simulink model "DFADAS2_SenFus_v1_201204RC_training_210115"  (R2018b)
settings: Solver=FixedStepDiscrete  StartTime=0.0  StopTime=inf  FixedStep=0.002  RelTol=1e-3  EnableMultiTasking=on
PreLoadFcn:
  | RTWConfigurationCB('preloadfcn', bdroot);
libraries: canmsglib x108, simulink x48, canfdmsglib x12
(part 3 of 28)

== system DFADAS2_SenFus_v1_201204RC_training_210115/Measure Calibration Debug/CAN Monitor (CANMon)/FLRdr ==
  <FLRdr> : Inport
  Bus Selector1 : BusSelector  OutputSignals=FLRdr_bsObjInfo.M00ObjInfo,FLRdr_bsObjInfo.M01ObjInfo,FLRdr_bsObjInfo.M10ObjInfo,FLRdr_bsObjInfo.M11ObjInfo
  Bus Selector2 : BusSelector  OutputSignals=Id_S0_003,XPos_S0_003,YPos_S0_003,XVelocity_S0_003,YVelocity_S0_003,XAcc_S0_003,YAcc_S0_003
  Bus Selector3 : BusSelector  OutputSignals=Id_S0_001,XPos_S0_001,YPos_S0_001,XVelocity_S0_001,YVelocity_S0_001,XAcc_S0_001,YAcc_S0_001
  Bus Selector4 : BusSelector  OutputSignals=Id_S0_002,XPos_S0_002,YPos_S0_002,XVelocity_S0_002,YVelocity_S0_002,XAcc_S0_002,YAcc_S0_002
  Bus Selector5 : BusSelector  OutputSignals=Id_S0_004,XPos_S0_004,YPos_S0_004,XVelocity_S0_004,YVelocity_S0_004,XAcc_S0_004,YAcc_S0_004
  CAN Pack1 : canmsglib/CAN Pack  MsgList=(none)  MsgName=CAN Msg  MsgIDType=Standard (11-bit identifier)  MsgIdentifier=2000  MsgLength=8  SignalInfo=ID$0$16$1$2$1$0$1$0$-Inf$Inf$#Xpos$16$16$1$2$1$0$0.05$-400$-Inf$Inf$#Ypos$32$16$1$2$1$0$0.01$-80$-Inf$Inf$#Vx$48$16$1$2$1$0$0.01$-80$-Inf$Inf$#  NSignals=4  StartBits=str2num('[int32(0);int32(16);int32(32);int32(48)]')  SignalSizes=str2num('[int32(16);int32(16);int32(16);int32(16)]')  ByteOrders=str2num('[int32(1);int32(1);int32(1);int32(1)]')  DataTypes=str2num('[int32(2);int32(2);int32(2);int32(2)]')  MultiplexTypes=str2num('[int32(1);int32(1);int32(1);int32(1)]')  MultiplexValues=str2num('[double(0);double(0);double(0);double(0)]')  Factors=str2num('[double(1);double(0.05);double(0.01);double(0.01)]')  Offsets=str2num('[double(0);double(-400);double(-80);double(-80)]')  Minimums=str2num('[double(-Inf);double(-Inf);double(-Inf);double(-Inf)]')  Maximums=str2num('[double(Inf);double(Inf);double(Inf);double(Inf)]')  Remote=off  ApplyMinMax=off  BusOutput=on
      settings: SourceProductName=Simulink Real-Time  SourceProductBaseCode=XP  DataFormat=manually specified signals
  CAN Pack2 : canmsglib/CAN Pack  MsgList=(none)  MsgName=CAN Msg  MsgIDType=Standard (11-bit identifier)  MsgIdentifier=2001  MsgLength=8  SignalInfo=VY$0$16$1$2$1$0$0.01$-80$-Inf$Inf$#Ax$16$16$1$2$1$0$0.01$-80$-Inf$Inf$#Ay$32$16$1$2$1$0$0.01$-80$-Inf$Inf$#singal$48$16$1$2$1$0$0.01$-80$-Inf$Inf$#  NSignals=4  StartBits=str2num('[int32(0);int32(16);int32(32);int32(48)]')  SignalSizes=str2num('[int32(16);int32(16);int32(16);int32(16)]')  ByteOrders=str2num('[int32(1);int32(1);int32(1);int32(1)]')  DataTypes=str2num('[int32(2);int32(2);int32(2);int32(2)]')  MultiplexTypes=str2num('[int32(1);int32(1);int32(1);int32(1)]')  MultiplexValues=str2num('[double(0);double(0);double(0);double(0)]')  Factors=str2num('[double(0.01);double(0.01);double(0.01);double(0.01)]')  Offsets=str2num('[double(-80);double(-80);double(-80);double(-80)]')  Minimums=str2num('[double(-Inf);double(-Inf);double(-Inf);double(-Inf)]')  Maximums=str2num('[double(Inf);double(Inf);double(Inf);double(Inf)]')  Remote=off  ApplyMinMax=off  BusOutput=on
      settings: SourceProductName=Simulink Real-Time  SourceProductBaseCode=XP  DataFormat=manually specified signals
  CAN Pack3 : canmsglib/CAN Pack  MsgList=(none)  MsgName=CAN Msg  MsgIDType=Standard (11-bit identifier)  MsgIdentifier=2002  MsgLength=8  SignalInfo=ID$0$16$1$2$1$0$1$0$-Inf$Inf$#Xpos$16$16$1$2$1$0$0.05$-400$-Inf$Inf$#Ypos$32$16$1$2$1$0$0.01$-80$-Inf$Inf$#Vx$48$16$1$2$1$0$0.01$-80$-Inf$Inf$#  NSignals=4  StartBits=str2num('[int32(0);int32(16);int32(32);int32(48)]')  SignalSizes=str2num('[int32(16);int32(16);int32(16);int32(16)]')  ByteOrders=str2num('[int32(1);int32(1);int32(1);int32(1)]')  DataTypes=str2num('[int32(2);int32(2);int32(2);int32(2)]')  MultiplexTypes=str2num('[int32(1);int32(1);int32(1);int32(1)]')  MultiplexValues=str2num('[double(0);double(0);double(0);double(0)]')  Factors=str2num('[double(1);double(0.05);double(0.01);double(0.01)]')  Offsets=str2num('[double(0);double(-400);double(-80);double(-80)]')  Minimums=str2num('[double(-Inf);double(-Inf);double(-Inf);double(-Inf)]')  Maximums=str2num('[double(Inf);double(Inf);double(Inf);double(Inf)]')  Remote=off  ApplyMinMax=off  BusOutput=on
      settings: SourceProductName=Simulink Real-Time  SourceProductBaseCode=XP  DataFormat=manually specified signals
  CAN Pack4 : canmsglib/CAN Pack  MsgList=(none)  MsgName=CAN Msg  MsgIDType=Standard (11-bit identifier)  MsgIdentifier=2003  MsgLength=8  SignalInfo=VY$0$16$1$2$1$0$0.01$-80$-Inf$Inf$#Ax$16$16$1$2$1$0$0.01$-80$-Inf$Inf$#Ay$32$16$1$2$1$0$0.01$-80$-Inf$Inf$#singal$48$16$1$2$1$0$0.01$-80$-Inf$Inf$#  NSignals=4  StartBits=str2num('[int32(0);int32(16);int32(32);int32(48)]')  SignalSizes=str2num('[int32(16);int32(16);int32(16);int32(16)]')  ByteOrders=str2num('[int32(1);int32(1);int32(1);int32(1)]')  DataTypes=str2num('[int32(2);int32(2);int32(2);int32(2)]')  MultiplexTypes=str2num('[int32(1);int32(1);int32(1);int32(1)]')  MultiplexValues=str2num('[double(0);double(0);double(0);double(0)]')  Factors=str2num('[double(0.01);double(0.01);double(0.01);double(0.01)]')  Offsets=str2num('[double(-80);double(-80);double(-80);double(-80)]')  Minimums=str2num('[double(-Inf);double(-Inf);double(-Inf);double(-Inf)]')  Maximums=str2num('[double(Inf);double(Inf);double(Inf);double(Inf)]')  Remote=off  ApplyMinMax=off  BusOutput=on
      settings: SourceProductName=Simulink Real-Time  SourceProductBaseCode=XP  DataFormat=manually specified signals
  CAN Pack5 : canmsglib/CAN Pack  MsgList=(none)  MsgName=CAN Msg  MsgIDType=Standard (11-bit identifier)  MsgIdentifier=2004  MsgLength=8  SignalInfo=ID$0$16$1$2$1$0$1$0$-Inf$Inf$#Xpos$16$16$1$2$1$0$0.05$-400$-Inf$Inf$#Ypos$32$16$1$2$1$0$0.01$-80$-Inf$Inf$#Vx$48$16$1$2$1$0$0.01$-80$-Inf$Inf$#  NSignals=4  StartBits=str2num('[int32(0);int32(16);int32(32);int32(48)]')  SignalSizes=str2num('[int32(16);int32(16);int32(16);int32(16)]')  ByteOrders=str2num('[int32(1);int32(1);int32(1);int32(1)]')  DataTypes=str2num('[int32(2);int32(2);int32(2);int32(2)]')  MultiplexTypes=str2num('[int32(1);int32(1);int32(1);int32(1)]')  MultiplexValues=str2num('[double(0);double(0);double(0);double(0)]')  Factors=str2num('[double(1);double(0.05);double(0.01);double(0.01)]')  Offsets=str2num('[double(0);double(-400);double(-80);double(-80)]')  Minimums=str2num('[double(-Inf);double(-Inf);double(-Inf);double(-Inf)]')  Maximums=str2num('[double(Inf);double(Inf);double(Inf);double(Inf)]')  Remote=off  ApplyMinMax=off  BusOutput=on
      settings: SourceProductName=Simulink Real-Time  SourceProductBaseCode=XP  DataFormat=manually specified signals
  CAN Pack6 : canmsglib/CAN Pack  MsgList=(none)  MsgName=CAN Msg  MsgIDType=Standard (11-bit identifier)  MsgIdentifier=2005  MsgLength=8  SignalInfo=VY$0$16$1$2$1$0$0.01$-80$-Inf$Inf$#Ax$16$16$1$2$1$0$0.01$-80$-Inf$Inf$#Ay$32$16$1$2$1$0$0.01$-80$-Inf$Inf$#singal$48$16$1$2$1$0$0.01$-80$-Inf$Inf$#  NSignals=4  StartBits=str2num('[int32(0);int32(16);int32(32);int32(48)]')  SignalSizes=str2num('[int32(16);int32(16);int32(16);int32(16)]')  ByteOrders=str2num('[int32(1);int32(1);int32(1);int32(1)]')  DataTypes=str2num('[int32(2);int32(2);int32(2);int32(2)]')  MultiplexTypes=str2num('[int32(1);int32(1);int32(1);int32(1)]')  MultiplexValues=str2num('[double(0);double(0);double(0);double(0)]')  Factors=str2num('[double(0.01);double(0.01);double(0.01);double(0.01)]')  Offsets=str2num('[double(-80);double(-80);double(-80);double(-80)]')  Minimums=str2num('[double(-Inf);double(-Inf);double(-Inf);double(-Inf)]')  Maximums=str2num('[double(Inf);double(Inf);double(Inf);double(Inf)]')  Remote=off  ApplyMinMax=off  BusOutput=on
      settings: SourceProductName=Simulink Real-Time  SourceProductBaseCode=XP  DataFormat=manually specified signals
  CAN Pack7 : canmsglib/CAN Pack  MsgList=(none)  MsgName=CAN Msg  MsgIDType=Standard (11-bit identifier)  MsgIdentifier=2006  MsgLength=8  SignalInfo=ID$0$16$1$2$1$0$1$0$-Inf$Inf$#Xpos$16$16$1$2$1$0$0.05$-400$-Inf$Inf$#Ypos$32$16$1$2$1$0$0.01$-80$-Inf$Inf$#Vx$48$16$1$2$1$0$0.01$-80$-Inf$Inf$#  NSignals=4  StartBits=str2num('[int32(0);int32(16);int32(32);int32(48)]')  SignalSizes=str2num('[int32(16);int32(16);int32(16);int32(16)]')  ByteOrders=str2num('[int32(1);int32(1);int32(1);int32(1)]')  DataTypes=str2num('[int32(2);int32(2);int32(2);int32(2)]')  MultiplexTypes=str2num('[int32(1);int32(1);int32(1);int32(1)]')  MultiplexValues=str2num('[double(0);double(0);double(0);double(0)]')  Factors=str2num('[double(1);double(0.05);double(0.01);double(0.01)]')  Offsets=str2num('[double(0);double(-400);double(-80);double(-80)]')  Minimums=str2num('[double(-Inf);double(-Inf);double(-Inf);double(-Inf)]')  Maximums=str2num('[double(Inf);double(Inf);double(Inf);double(Inf)]')  Remote=off  ApplyMinMax=off  BusOutput=on
      settings: SourceProductName=Simulink Real-Time  SourceProductBaseCode=XP  DataFormat=manually specified signals
  CAN Pack8 : canmsglib/CAN Pack  MsgList=(none)  MsgName=CAN Msg  MsgIDType=Standard (11-bit identifier)  MsgIdentifier=2007  MsgLength=8  SignalInfo=VY$0$16$1$2$1$0$0.01$-80$-Inf$Inf$#Ax$16$16$1$2$1$0$0.01$-80$-Inf$Inf$#Ay$32$16$1$2$1$0$0.01$-80$-Inf$Inf$#singal$48$16$1$2$1$0$0.01$-80$-Inf$Inf$#  NSignals=4  StartBits=str2num('[int32(0);int32(16);int32(32);int32(48)]')  SignalSizes=str2num('[int32(16);int32(16);int32(16);int32(16)]')  ByteOrders=str2num('[int32(1);int32(1);int32(1);int32(1)]')  DataTypes=str2num('[int32(2);int32(2);int32(2);int32(2)]')  MultiplexTypes=str2num('[int32(1);int32(1);int32(1);int32(1)]')  MultiplexValues=str2num('[double(0);double(0);double(0);double(0)]')  Factors=str2num('[double(0.01);double(0.01);double(0.01);double(0.01)]')  Offsets=str2num('[double(-80);double(-80);double(-80);double(-80)]')  Minimums=str2num('[double(-Inf);double(-Inf);double(-Inf);double(-Inf)]')  Maximums=str2num('[double(Inf);double(Inf);double(Inf);double(Inf)]')  Remote=off  ApplyMinMax=off  BusOutput=on
      settings: SourceProductName=Simulink Real-Time  SourceProductBaseCode=XP  DataFormat=manually specified signals
  S-Function1 : S-Function  FunctionName=NSTC297CANTransmitBlkLib  Parameters=|  SFunctionDeploymentMode=off  EnableBusSupport=off  mask(NSTC297 CAN Transmit){Ns_DeviceID=General Control Unit Gen2, Ns_ChannelNum=0, Ns_FrameType=CAN, Ns_FrameBufferSize=0, Ns_OverflowCntOutFlg=off, Ns_SampleTime=-1}
      | uint16(Ns_DeviceID),
      | uint16(Ns_ChannelNum),
      | uint16(Ns_FrameType),
      | uint16(Ns_FrameBufferSize),
      | uint8(Ns_OverflowCntOutFlg),
      | double(Ns_SampleTime)
      mask prompts: Ns_DeviceID "Device:"; Ns_ChannelNum "Channel number:"; Ns_FrameType "Frame type:"; Ns_FrameBufferSize "Frame buffer size:"; Ns_OverflowCntOutFlg "Overflow count output"; Ns_SampleTime "Sample time:"
      mask init:
      | NSTC297CANTransmit_callback('portlabels');
      mask TypeOptions Ns_DeviceID: General Control Unit Gen2 | ADAS Control Unit Gen2
      mask TypeOptions Ns_ChannelNum: 0 | 1 | 2 | 3 | 4 | 5
      mask TypeOptions Ns_FrameType: CAN | CANFD
      mask Display: color('blue');text(0.98,0.9,'NovSteeds TC297','horizontalAlignment','right');color('blue');text(0.5,0.65,'CAN Transmit','horizontalAlignment','center');color('black');text(0.5,0.35,'Type: CAN','horizontalAlignment','center');text(0.5,0.50,'Channel: 0','horizontalAlignment','center');port_label('input',1, 'Msg');
  S-Function2 : S-Function  FunctionName=NSTC297CANTransmitBlkLib  Parameters=|  SFunctionDeploymentMode=off  EnableBusSupport=off  mask(NSTC297 CAN Transmit){Ns_DeviceID=General Control Unit Gen2, Ns_ChannelNum=0, Ns_FrameType=CAN, Ns_FrameBufferSize=0, Ns_OverflowCntOutFlg=off, Ns_SampleTime=-1}
      | uint16(Ns_DeviceID),
      | uint16(Ns_ChannelNum),
      | uint16(Ns_FrameType),
      | uint16(Ns_FrameBufferSize),
      | uint8(Ns_OverflowCntOutFlg),
      | double(Ns_SampleTime)
      mask prompts: Ns_DeviceID "Device:"; Ns_ChannelNum "Channel number:"; Ns_FrameType "Frame type:"; Ns_FrameBufferSize "Frame buffer size:"; Ns_OverflowCntOutFlg "Overflow count output"; Ns_SampleTime "Sample time:"
      mask init:
      | NSTC297CANTransmit_callback('portlabels');
      mask TypeOptions Ns_DeviceID: General Control Unit Gen2 | ADAS Control Unit Gen2
      mask TypeOptions Ns_ChannelNum: 0 | 1 | 2 | 3 | 4 | 5
      mask TypeOptions Ns_FrameType: CAN | CANFD
      mask Display: color('blue');text(0.98,0.9,'NovSteeds TC297','horizontalAlignment','right');color('blue');text(0.5,0.65,'CAN Transmit','horizontalAlignment','center');color('black');text(0.5,0.35,'Type: CAN','horizontalAlignment','center');text(0.5,0.50,'Channel: 0','horizontalAlignment','center');port_label('input',1, 'Msg');
  S-Function3 : S-Function  FunctionName=NSTC297CANTransmitBlkLib  Parameters=|  SFunctionDeploymentMode=off  EnableBusSupport=off  mask(NSTC297 CAN Transmit){Ns_DeviceID=General Control Unit Gen2, Ns_ChannelNum=0, Ns_FrameType=CAN, Ns_FrameBufferSize=0, Ns_OverflowCntOutFlg=off, Ns_SampleTime=-1}
      | uint16(Ns_DeviceID),
      | uint16(Ns_ChannelNum),
      | uint16(Ns_FrameType),
      | uint16(Ns_FrameBufferSize),
      | uint8(Ns_OverflowCntOutFlg),
      | double(Ns_SampleTime)
      mask prompts: Ns_DeviceID "Device:"; Ns_ChannelNum "Channel number:"; Ns_FrameType "Frame type:"; Ns_FrameBufferSize "Frame buffer size:"; Ns_OverflowCntOutFlg "Overflow count output"; Ns_SampleTime "Sample time:"
      mask init:
      | NSTC297CANTransmit_callback('portlabels');
      mask TypeOptions Ns_DeviceID: General Control Unit Gen2 | ADAS Control Unit Gen2
      mask TypeOptions Ns_ChannelNum: 0 | 1 | 2 | 3 | 4 | 5
      mask TypeOptions Ns_FrameType: CAN | CANFD
      mask Display: color('blue');text(0.98,0.9,'NovSteeds TC297','horizontalAlignment','right');color('blue');text(0.5,0.65,'CAN Transmit','horizontalAlignment','center');color('black');text(0.5,0.35,'Type: CAN','horizontalAlignment','center');text(0.5,0.50,'Channel: 0','horizontalAlignment','center');port_label('input',1, 'Msg');
  S-Function4 : S-Function  FunctionName=NSTC297CANTransmitBlkLib  Parameters=|  SFunctionDeploymentMode=off  EnableBusSupport=off  mask(NSTC297 CAN Transmit){Ns_DeviceID=General Control Unit Gen2, Ns_ChannelNum=0, Ns_FrameType=CAN, Ns_FrameBufferSize=0, Ns_OverflowCntOutFlg=off, Ns_SampleTime=-1}
      | uint16(Ns_DeviceID),
      | uint16(Ns_ChannelNum),
      | uint16(Ns_FrameType),
      | uint16(Ns_FrameBufferSize),
      | uint8(Ns_OverflowCntOutFlg),
      | double(Ns_SampleTime)
      mask prompts: Ns_DeviceID "Device:"; Ns_ChannelNum "Channel number:"; Ns_FrameType "Frame type:"; Ns_FrameBufferSize "Frame buffer size:"; Ns_OverflowCntOutFlg "Overflow count output"; Ns_SampleTime "Sample time:"
      mask init:
      | NSTC297CANTransmit_callback('portlabels');
      mask TypeOptions Ns_DeviceID: General Control Unit Gen2 | ADAS Control Unit Gen2
      mask TypeOptions Ns_ChannelNum: 0 | 1 | 2 | 3 | 4 | 5
      mask TypeOptions Ns_FrameType: CAN | CANFD
      mask Display: color('blue');text(0.98,0.9,'NovSteeds TC297','horizontalAlignment','right');color('blue');text(0.5,0.65,'CAN Transmit','horizontalAlignment','center');color('black');text(0.5,0.35,'Type: CAN','horizontalAlignment','center');text(0.5,0.50,'Channel: 0','horizontalAlignment','center');port_label('input',1, 'Msg');
  S-Function5 : S-Function  FunctionName=NSTC297CANTransmitBlkLib  Parameters=|  SFunctionDeploymentMode=off  EnableBusSupport=off  mask(NSTC297 CAN Transmit){Ns_DeviceID=General Control Unit Gen2, Ns_ChannelNum=0, Ns_FrameType=CAN, Ns_FrameBufferSize=0, Ns_OverflowCntOutFlg=off, Ns_SampleTime=-1}
      | uint16(Ns_DeviceID),
      | uint16(Ns_ChannelNum),
      | uint16(Ns_FrameType),
      | uint16(Ns_FrameBufferSize),
      | uint8(Ns_OverflowCntOutFlg),
      | double(Ns_SampleTime)
      mask prompts: Ns_DeviceID "Device:"; Ns_ChannelNum "Channel number:"; Ns_FrameType "Frame type:"; Ns_FrameBufferSize "Frame buffer size:"; Ns_OverflowCntOutFlg "Overflow count output"; Ns_SampleTime "Sample time:"
      mask init:
      | NSTC297CANTransmit_callback('portlabels');
      mask TypeOptions Ns_DeviceID: General Control Unit Gen2 | ADAS Control Unit Gen2
      mask TypeOptions Ns_ChannelNum: 0 | 1 | 2 | 3 | 4 | 5
      mask TypeOptions Ns_FrameType: CAN | CANFD
      mask Display: color('blue');text(0.98,0.9,'NovSteeds TC297','horizontalAlignment','right');color('blue');text(0.5,0.65,'CAN Transmit','horizontalAlignment','center');color('black');text(0.5,0.35,'Type: CAN','horizontalAlignment','center');text(0.5,0.50,'Channel: 0','horizontalAlignment','center');port_label('input',1, 'Msg');
  S-Function6 : S-Function  FunctionName=NSTC297CANTransmitBlkLib  Parameters=|  SFunctionDeploymentMode=off  EnableBusSupport=off  mask(NSTC297 CAN Transmit){Ns_DeviceID=General Control Unit Gen2, Ns_ChannelNum=0, Ns_FrameType=CAN, Ns_FrameBufferSize=0, Ns_OverflowCntOutFlg=off, Ns_SampleTime=-1}
      | uint16(Ns_DeviceID),
      | uint16(Ns_ChannelNum),
      | uint16(Ns_FrameType),
      | uint16(Ns_FrameBufferSize),
      | uint8(Ns_OverflowCntOutFlg),
      | double(Ns_SampleTime)
      mask prompts: Ns_DeviceID "Device:"; Ns_ChannelNum "Channel number:"; Ns_FrameType "Frame type:"; Ns_FrameBufferSize "Frame buffer size:"; Ns_OverflowCntOutFlg "Overflow count output"; Ns_SampleTime "Sample time:"
      mask init:
      | NSTC297CANTransmit_callback('portlabels');
      mask TypeOptions Ns_DeviceID: General Control Unit Gen2 | ADAS Control Unit Gen2
      mask TypeOptions Ns_ChannelNum: 0 | 1 | 2 | 3 | 4 | 5
      mask TypeOptions Ns_FrameType: CAN | CANFD
      mask Display: color('blue');text(0.98,0.9,'NovSteeds TC297','horizontalAlignment','right');color('blue');text(0.5,0.65,'CAN Transmit','horizontalAlignment','center');color('black');text(0.5,0.35,'Type: CAN','horizontalAlignment','center');text(0.5,0.50,'Channel: 0','horizontalAlignment','center');port_label('input',1, 'Msg');
  S-Function7 : S-Function  FunctionName=NSTC297CANTransmitBlkLib  Parameters=|  SFunctionDeploymentMode=off  EnableBusSupport=off  mask(NSTC297 CAN Transmit){Ns_DeviceID=General Control Unit Gen2, Ns_ChannelNum=0, Ns_FrameType=CAN, Ns_FrameBufferSize=0, Ns_OverflowCntOutFlg=off, Ns_SampleTime=-1}
      | uint16(Ns_DeviceID),
      | uint16(Ns_ChannelNum),
      | uint16(Ns_FrameType),
      | uint16(Ns_FrameBufferSize),
      | uint8(Ns_OverflowCntOutFlg),
      | double(Ns_SampleTime)
      mask prompts: Ns_DeviceID "Device:"; Ns_ChannelNum "Channel number:"; Ns_FrameType "Frame type:"; Ns_FrameBufferSize "Frame buffer size:"; Ns_OverflowCntOutFlg "Overflow count output"; Ns_SampleTime "Sample time:"
      mask init:
      | NSTC297CANTransmit_callback('portlabels');
      mask TypeOptions Ns_DeviceID: General Control Unit Gen2 | ADAS Control Unit Gen2
      mask TypeOptions Ns_ChannelNum: 0 | 1 | 2 | 3 | 4 | 5
      mask TypeOptions Ns_FrameType: CAN | CANFD
      mask Display: color('blue');text(0.98,0.9,'NovSteeds TC297','horizontalAlignment','right');color('blue');text(0.5,0.65,'CAN Transmit','horizontalAlignment','center');color('black');text(0.5,0.35,'Type: CAN','horizontalAlignment','center');text(0.5,0.50,'Channel: 0','horizontalAlignment','center');port_label('input',1, 'Msg');
  S-Function8 : S-Function  FunctionName=NSTC297CANTransmitBlkLib  Parameters=|  SFunctionDeploymentMode=off  EnableBusSupport=off  mask(NSTC297 CAN Transmit){Ns_DeviceID=General Control Unit Gen2, Ns_ChannelNum=0, Ns_FrameType=CAN, Ns_FrameBufferSize=0, Ns_OverflowCntOutFlg=off, Ns_SampleTime=-1}
      | uint16(Ns_DeviceID),
      | uint16(Ns_ChannelNum),
      | uint16(Ns_FrameType),
      | uint16(Ns_FrameBufferSize),
      | uint8(Ns_OverflowCntOutFlg),
      | double(Ns_SampleTime)
      mask prompts: Ns_DeviceID "Device:"; Ns_ChannelNum "Channel number:"; Ns_FrameType "Frame type:"; Ns_FrameBufferSize "Frame buffer size:"; Ns_OverflowCntOutFlg "Overflow count output"; Ns_SampleTime "Sample time:"
      mask init:
      | NSTC297CANTransmit_callback('portlabels');
      mask TypeOptions Ns_DeviceID: General Control Unit Gen2 | ADAS Control Unit Gen2
      mask TypeOptions Ns_ChannelNum: 0 | 1 | 2 | 3 | 4 | 5
      mask TypeOptions Ns_FrameType: CAN | CANFD
      mask Display: color('blue');text(0.98,0.9,'NovSteeds TC297','horizontalAlignment','right');color('blue');text(0.5,0.65,'CAN Transmit','horizontalAlignment','center');color('black');text(0.5,0.35,'Type: CAN','horizontalAlignment','center');text(0.5,0.50,'Channel: 0','horizontalAlignment','center');port_label('input',1, 'Msg');
  wires:
  Bus Selector1/1 -> Bus Selector3/1  "<M00ObjInfo>"
  Bus Selector1/2 -> Bus Selector4/1  "<M01ObjInfo>"
  Bus Selector1/4 -> Bus Selector5/1  "<M11ObjInfo>"
  Bus Selector1/3 -> Bus Selector2/1  "<M10ObjInfo>"
  <FLRdr>/1 -> Bus Selector1/1
  CAN Pack1/1 -> S-Function8/1
  CAN Pack2/1 -> S-Function1/1
  Bus Selector3/5 -> CAN Pack2/1  "<YVelocity_S0_001>"
  Bus Selector3/6 -> CAN Pack2/2  "<XAcc_S0_001>"
  Bus Selector3/7 -> CAN Pack2/3  "<YAcc_S0_001>"
  Bus Selector3/1 -> CAN Pack1/1  "<Id_S0_001>"
  Bus Selector3/2 -> CAN Pack1/2  "<XPos_S0_001>"
  Bus Selector3/3 -> CAN Pack1/3  "<YPos_S0_001>"
  Bus Selector3/4 -> CAN Pack1/4  "<XVelocity_S0_001>"
  Bus Selector4/4 -> CAN Pack3/4  "<XVelocity_S0_002>"
  Bus Selector4/3 -> CAN Pack3/3  "<YPos_S0_002>"
  Bus Selector4/2 -> CAN Pack3/2  "<XPos_S0_002>"
  Bus Selector4/1 -> CAN Pack3/1  "<Id_S0_002>"
  Bus Selector4/7 -> CAN Pack4/3  "<YAcc_S0_002>"
  Bus Selector4/6 -> CAN Pack4/2  "<XAcc_S0_002>"
  Bus Selector4/5 -> CAN Pack4/1  "<YVelocity_S0_002>"
  CAN Pack4/1 -> S-Function2/1
  CAN Pack3/1 -> S-Function3/1
  CAN Pack5/1 -> S-Function5/1
  CAN Pack6/1 -> S-Function4/1
  Bus Selector2/5 -> CAN Pack6/1  "<YVelocity_S0_003>"
  Bus Selector2/6 -> CAN Pack6/2  "<XAcc_S0_003>"
  Bus Selector2/7 -> CAN Pack6/3  "<YAcc_S0_003>"
  Bus Selector2/1 -> CAN Pack5/1  "<Id_S0_003>"
  Bus Selector2/2 -> CAN Pack5/2  "<XPos_S0_003>"
  Bus Selector2/3 -> CAN Pack5/3  "<YPos_S0_003>"
  Bus Selector2/4 -> CAN Pack5/4  "<XVelocity_S0_003>"
  Bus Selector5/4 -> CAN Pack7/4  "<XVelocity_S0_004>"
  Bus Selector5/3 -> CAN Pack7/3  "<YPos_S0_004>"
  Bus Selector5/2 -> CAN Pack7/2  "<XPos_S0_004>"
  Bus Selector5/7 -> CAN Pack8/3  "<YAcc_S0_004>"
  Bus Selector5/6 -> CAN Pack8/2  "<XAcc_S0_004>"
  Bus Selector5/5 -> CAN Pack8/1  "<YVelocity_S0_004>"
  CAN Pack8/1 -> S-Function6/1
  CAN Pack7/1 -> S-Function7/1
  Bus Selector5/1 -> CAN Pack7/1  "<Id_S0_004>"

== system DFADAS2_SenFus_v1_201204RC_training_210115/Measure Calibration Debug/CAN Monitor (CANMon)/FRRdr ==
  <FRRdr> : Inport
  Bus Selector1 : BusSelector  OutputSignals=FRRdr_bsObjInfo.M00ObjInfo,FRRdr_bsObjInfo.M01ObjInfo,FRRdr_bsObjInfo.M10ObjInfo,FRRdr_bsObjInfo.M11ObjInfo
  Bus Selector2 : BusSelector  OutputSignals=Id_S0_003,XPos_S0_003,YPos_S0_003,XVelocity_S0_003,YVelocity_S0_003,XAcc_S0_003,YAcc_S0_003
  Bus Selector3 : BusSelector  OutputSignals=Id_S0_001,XPos_S0_001,YPos_S0_001,XVelocity_S0_001,YVelocity_S0_001,XAcc_S0_001,YAcc_S0_001
  Bus Selector4 : BusSelector  OutputSignals=Id_S0_002,XPos_S0_002,YPos_S0_002,XVelocity_S0_002,YVelocity_S0_002,XAcc_S0_002,YAcc_S0_002
  Bus Selector5 : BusSelector  OutputSignals=Id_S0_004,XPos_S0_004,YPos_S0_004,XVelocity_S0_004,YVelocity_S0_004,XAcc_S0_004,YAcc_S0_004
  CAN Pack1 : canmsglib/CAN Pack  MsgList=(none)  MsgName=CAN Msg  MsgIDType=Standard (11-bit identifier)  MsgIdentifier=2008  MsgLength=8  SignalInfo=ID$0$16$1$2$1$0$1$0$-Inf$Inf$#Xpos$16$16$1$2$1$0$0.05$-400$-Inf$Inf$#Ypos$32$16$1$2$1$0$0.01$-80$-Inf$Inf$#Vx$48$16$1$2$1$0$0.01$-80$-Inf$Inf$#  NSignals=4  StartBits=str2num('[int32(0);int32(16);int32(32);int32(48)]')  SignalSizes=str2num('[int32(16);int32(16);int32(16);int32(16)]')  ByteOrders=str2num('[int32(1);int32(1);int32(1);int32(1)]')  DataTypes=str2num('[int32(2);int32(2);int32(2);int32(2)]')  MultiplexTypes=str2num('[int32(1);int32(1);int32(1);int32(1)]')  MultiplexValues=str2num('[double(0);double(0);double(0);double(0)]')  Factors=str2num('[double(1);double(0.05);double(0.01);double(0.01)]')  Offsets=str2num('[double(0);double(-400);double(-80);double(-80)]')  Minimums=str2num('[double(-Inf);double(-Inf);double(-Inf);double(-Inf)]')  Maximums=str2num('[double(Inf);double(Inf);double(Inf);double(Inf)]')  Remote=off  ApplyMinMax=off  BusOutput=on
      settings: SourceProductName=Simulink Real-Time  SourceProductBaseCode=XP  DataFormat=manually specified signals
  CAN Pack10 : canmsglib/CAN Pack  MsgList=(none)  MsgName=CAN Msg  MsgIDType=Standard (11-bit identifier)  MsgIdentifier=2015  MsgLength=8  SignalInfo=VY$0$16$1$2$1$0$0.01$-80$-Inf$Inf$#Ax$16$16$1$2$1$0$0.01$-80$-Inf$Inf$#Ay$32$16$1$2$1$0$0.01$-80$-Inf$Inf$#singal$48$16$1$2$1$0$0.01$-80$-Inf$Inf$#  NSignals=4  StartBits=str2num('[int32(0);int32(16);int32(32);int32(48)]')  SignalSizes=str2num('[int32(16);int32(16);int32(16);int32(16)]')  ByteOrders=str2num('[int32(1);int32(1);int32(1);int32(1)]')  DataTypes=str2num('[int32(2);int32(2);int32(2);int32(2)]')  MultiplexTypes=str2num('[int32(1);int32(1);int32(1);int32(1)]')  MultiplexValues=str2num('[double(0);double(0);double(0);double(0)]')  Factors=str2num('[double(0.01);double(0.01);double(0.01);double(0.01)]')  Offsets=str2num('[double(-80);double(-80);double(-80);double(-80)]')  Minimums=str2num('[double(-Inf);double(-Inf);double(-Inf);double(-Inf)]')  Maximums=str2num('[double(Inf);double(Inf);double(Inf);double(Inf)]')  Remote=off  ApplyMinMax=off  BusOutput=on
      settings: SourceProductName=Simulink Real-Time  SourceProductBaseCode=XP  DataFormat=manually specified signals
  CAN Pack2 : canmsglib/CAN Pack  MsgList=(none)  MsgName=CAN Msg  MsgIDType=Standard (11-bit identifier)  MsgIdentifier=2009  MsgLength=8  SignalInfo=VY$0$16$1$2$1$0$0.01$-80$-Inf$Inf$#Ax$16$16$1$2$1$0$0.01$-80$-Inf$Inf$#Ay$32$16$1$2$1$0$0.01$-80$-Inf$Inf$#singal$48$16$1$2$1$0$0.01$-80$-Inf$Inf$#  NSignals=4  StartBits=str2num('[int32(0);int32(16);int32(32);int32(48)]')  SignalSizes=str2num('[int32(16);int32(16);int32(16);int32(16)]')  ByteOrders=str2num('[int32(1);int32(1);int32(1);int32(1)]')  DataTypes=str2num('[int32(2);int32(2);int32(2);int32(2)]')  MultiplexTypes=str2num('[int32(1);int32(1);int32(1);int32(1)]')  MultiplexValues=str2num('[double(0);double(0);double(0);double(0)]')  Factors=str2num('[double(0.01);double(0.01);double(0.01);double(0.01)]')  Offsets=str2num('[double(-80);double(-80);double(-80);double(-80)]')  Minimums=str2num('[double(-Inf);double(-Inf);double(-Inf);double(-Inf)]')  Maximums=str2num('[double(Inf);double(Inf);double(Inf);double(Inf)]')  Remote=off  ApplyMinMax=off  BusOutput=on
      settings: SourceProductName=Simulink Real-Time  SourceProductBaseCode=XP  DataFormat=manually specified signals
  CAN Pack3 : canmsglib/CAN Pack  MsgList=(none)  MsgName=CAN Msg  MsgIDType=Standard (11-bit identifier)  MsgIdentifier=2010  MsgLength=8  SignalInfo=ID$0$16$1$2$1$0$1$0$-Inf$Inf$#Xpos$16$16$1$2$1$0$0.05$-400$-Inf$Inf$#Ypos$32$16$1$2$1$0$0.01$-80$-Inf$Inf$#Vx$48$16$1$2$1$0$0.01$-80$-Inf$Inf$#  NSignals=4  StartBits=str2num('[int32(0);int32(16);int32(32);int32(48)]')  SignalSizes=str2num('[int32(16);int32(16);int32(16);int32(16)]')  ByteOrders=str2num('[int32(1);int32(1);int32(1);int32(1)]')  DataTypes=str2num('[int32(2);int32(2);int32(2);int32(2)]')  MultiplexTypes=str2num('[int32(1);int32(1);int32(1);int32(1)]')  MultiplexValues=str2num('[double(0);double(0);double(0);double(0)]')  Factors=str2num('[double(1);double(0.05);double(0.01);double(0.01)]')  Offsets=str2num('[double(0);double(-400);double(-80);double(-80)]')  Minimums=str2num('[double(-Inf);double(-Inf);double(-Inf);double(-Inf)]')  Maximums=str2num('[double(Inf);double(Inf);double(Inf);double(Inf)]')  Remote=off  ApplyMinMax=off  BusOutput=on
      settings: SourceProductName=Simulink Real-Time  SourceProductBaseCode=XP  DataFormat=manually specified signals
  CAN Pack4 : canmsglib/CAN Pack  MsgList=(none)  MsgName=CAN Msg  MsgIDType=Standard (11-bit identifier)  MsgIdentifier=2011  MsgLength=8  SignalInfo=VY$0$16$1$2$1$0$0.01$-80$-Inf$Inf$#Ax$16$16$1$2$1$0$0.01$-80$-Inf$Inf$#Ay$32$16$1$2$1$0$0.01$-80$-Inf$Inf$#singal$48$16$1$2$1$0$0.01$-80$-Inf$Inf$#  NSignals=4  StartBits=str2num('[int32(0);int32(16);int32(32);int32(48)]')  SignalSizes=str2num('[int32(16);int32(16);int32(16);int32(16)]')  ByteOrders=str2num('[int32(1);int32(1);int32(1);int32(1)]')  DataTypes=str2num('[int32(2);int32(2);int32(2);int32(2)]')  MultiplexTypes=str2num('[int32(1);int32(1);int32(1);int32(1)]')  MultiplexValues=str2num('[double(0);double(0);double(0);double(0)]')  Factors=str2num('[double(0.01);double(0.01);double(0.01);double(0.01)]')  Offsets=str2num('[double(-80);double(-80);double(-80);double(-80)]')  Minimums=str2num('[double(-Inf);double(-Inf);double(-Inf);double(-Inf)]')  Maximums=str2num('[double(Inf);double(Inf);double(Inf);double(Inf)]')  Remote=off  ApplyMinMax=off  BusOutput=on
      settings: SourceProductName=Simulink Real-Time  SourceProductBaseCode=XP  DataFormat=manually specified signals
  CAN Pack5 : canmsglib/CAN Pack  MsgList=(none)  MsgName=CAN Msg  MsgIDType=Standard (11-bit identifier)  MsgIdentifier=2012  MsgLength=8  SignalInfo=ID$0$16$1$2$1$0$1$0$-Inf$Inf$#Xpos$16$16$1$2$1$0$0.05$-400$-Inf$Inf$#Ypos$32$16$1$2$1$0$0.01$-80$-Inf$Inf$#Vx$48$16$1$2$1$0$0.01$-80$-Inf$Inf$#  NSignals=4  StartBits=str2num('[int32(0);int32(16);int32(32);int32(48)]')  SignalSizes=str2num('[int32(16);int32(16);int32(16);int32(16)]')  ByteOrders=str2num('[int32(1);int32(1);int32(1);int32(1)]')  DataTypes=str2num('[int32(2);int32(2);int32(2);int32(2)]')  MultiplexTypes=str2num('[int32(1);int32(1);int32(1);int32(1)]')  MultiplexValues=str2num('[double(0);double(0);double(0);double(0)]')  Factors=str2num('[double(1);double(0.05);double(0.01);double(0.01)]')  Offsets=str2num('[double(0);double(-400);double(-80);double(-80)]')  Minimums=str2num('[double(-Inf);double(-Inf);double(-Inf);double(-Inf)]')  Maximums=str2num('[double(Inf);double(Inf);double(Inf);double(Inf)]')  Remote=off  ApplyMinMax=off  BusOutput=on
      settings: SourceProductName=Simulink Real-Time  SourceProductBaseCode=XP  DataFormat=manually specified signals
  CAN Pack6 : canmsglib/CAN Pack  MsgList=(none)  MsgName=CAN Msg  MsgIDType=Standard (11-bit identifier)  MsgIdentifier=2013  MsgLength=8  SignalInfo=VY$0$16$1$2$1$0$0.01$-80$-Inf$Inf$#Ax$16$16$1$2$1$0$0.01$-80$-Inf$Inf$#Ay$32$16$1$2$1$0$0.01$-80$-Inf$Inf$#singal$48$16$1$2$1$0$0.01$-80$-Inf$Inf$#  NSignals=4  StartBits=str2num('[int32(0);int32(16);int32(32);int32(48)]')  SignalSizes=str2num('[int32(16);int32(16);int32(16);int32(16)]')  ByteOrders=str2num('[int32(1);int32(1);int32(1);int32(1)]')  DataTypes=str2num('[int32(2);int32(2);int32(2);int32(2)]')  MultiplexTypes=str2num('[int32(1);int32(1);int32(1);int32(1)]')  MultiplexValues=str2num('[double(0);double(0);double(0);double(0)]')  Factors=str2num('[double(0.01);double(0.01);double(0.01);double(0.01)]')  Offsets=str2num('[double(-80);double(-80);double(-80);double(-80)]')  Minimums=str2num('[double(-Inf);double(-Inf);double(-Inf);double(-Inf)]')  Maximums=str2num('[double(Inf);double(Inf);double(Inf);double(Inf)]')  Remote=off  ApplyMinMax=off  BusOutput=on
      settings: SourceProductName=Simulink Real-Time  SourceProductBaseCode=XP  DataFormat=manually specified signals
  CAN Pack9 : canmsglib/CAN Pack  MsgList=(none)  MsgName=CAN Msg  MsgIDType=Standard (11-bit identifier)  MsgIdentifier=2014  MsgLength=8  SignalInfo=ID$0$16$1$2$1$0$1$0$-Inf$Inf$#Xpos$16$16$1$2$1$0$0.05$-400$-Inf$Inf$#Ypos$32$16$1$2$1$0$0.01$-80$-Inf$Inf$#Vx$48$16$1$2$1$0$0.01$-80$-Inf$Inf$#  NSignals=4  StartBits=str2num('[int32(0);int32(16);int32(32);int32(48)]')  SignalSizes=str2num('[int32(16);int32(16);int32(16);int32(16)]')  ByteOrders=str2num('[int32(1);int32(1);int32(1);int32(1)]')  DataTypes=str2num('[int32(2);int32(2);int32(2);int32(2)]')  MultiplexTypes=str2num('[int32(1);int32(1);int32(1);int32(1)]')  MultiplexValues=str2num('[double(0);double(0);double(0);double(0)]')  Factors=str2num('[double(1);double(0.05);double(0.01);double(0.01)]')  Offsets=str2num('[double(0);double(-400);double(-80);double(-80)]')  Minimums=str2num('[double(-Inf);double(-Inf);double(-Inf);double(-Inf)]')  Maximums=str2num('[double(Inf);double(Inf);double(Inf);double(Inf)]')  Remote=off  ApplyMinMax=off  BusOutput=on
      settings: SourceProductName=Simulink Real-Time  SourceProductBaseCode=XP  DataFormat=manually specified signals
  S-Function1 : S-Function  FunctionName=NSTC297CANTransmitBlkLib  Parameters=|  SFunctionDeploymentMode=off  EnableBusSupport=off  mask(NSTC297 CAN Transmit){Ns_DeviceID=General Control Unit Gen2, Ns_ChannelNum=0, Ns_FrameType=CAN, Ns_FrameBufferSize=0, Ns_OverflowCntOutFlg=off, Ns_SampleTime=-1}
      | uint16(Ns_DeviceID),
      | uint16(Ns_ChannelNum),
      | uint16(Ns_FrameType),
      | uint16(Ns_FrameBufferSize),
      | uint8(Ns_OverflowCntOutFlg),
      | double(Ns_SampleTime)
      mask prompts: Ns_DeviceID "Device:"; Ns_ChannelNum "Channel number:"; Ns_FrameType "Frame type:"; Ns_FrameBufferSize "Frame buffer size:"; Ns_OverflowCntOutFlg "Overflow count output"; Ns_SampleTime "Sample time:"
      mask init:
      | NSTC297CANTransmit_callback('portlabels');
      mask TypeOptions Ns_DeviceID: General Control Unit Gen2 | ADAS Control Unit Gen2
      mask TypeOptions Ns_ChannelNum: 0 | 1 | 2 | 3 | 4 | 5
      mask TypeOptions Ns_FrameType: CAN | CANFD
      mask Display: color('blue');text(0.98,0.9,'NovSteeds TC297','horizontalAlignment','right');color('blue');text(0.5,0.65,'CAN Transmit','horizontalAlignment','center');color('black');text(0.5,0.35,'Type: CAN','horizontalAlignment','center');text(0.5,0.50,'Channel: 0','horizontalAlignment','center');port_label('input',1, 'Msg');
  S-Function10 : S-Function  FunctionName=NSTC297CANTransmitBlkLib  Parameters=|  SFunctionDeploymentMode=off  EnableBusSupport=off  mask(NSTC297 CAN Transmit){Ns_DeviceID=General Control Unit Gen2, Ns_ChannelNum=0, Ns_FrameType=CAN, Ns_FrameBufferSize=0, Ns_OverflowCntOutFlg=off, Ns_SampleTime=-1}
      | uint16(Ns_DeviceID),
      | uint16(Ns_ChannelNum),
      | uint16(Ns_FrameType),
      | uint16(Ns_FrameBufferSize),
      | uint8(Ns_OverflowCntOutFlg),
      | double(Ns_SampleTime)
      mask prompts: Ns_DeviceID "Device:"; Ns_ChannelNum "Channel number:"; Ns_FrameType "Frame type:"; Ns_FrameBufferSize "Frame buffer size:"; Ns_OverflowCntOutFlg "Overflow count output"; Ns_SampleTime "Sample time:"
      mask init:
      | NSTC297CANTransmit_callback('portlabels');
      mask TypeOptions Ns_DeviceID: General Control Unit Gen2 | ADAS Control Unit Gen2
      mask TypeOptions Ns_ChannelNum: 0 | 1 | 2 | 3 | 4 | 5
      mask TypeOptions Ns_FrameType: CAN | CANFD
      mask Display: color('blue');text(0.98,0.9,'NovSteeds TC297','horizontalAlignment','right');color('blue');text(0.5,0.65,'CAN Transmit','horizontalAlignment','center');color('black');text(0.5,0.35,'Type: CAN','horizontalAlignment','center');text(0.5,0.50,'Channel: 0','horizontalAlignment','center');port_label('input',1, 'Msg');
  S-Function2 : S-Function  FunctionName=NSTC297CANTransmitBlkLib  Parameters=|  SFunctionDeploymentMode=off  EnableBusSupport=off  mask(NSTC297 CAN Transmit){Ns_DeviceID=General Control Unit Gen2, Ns_ChannelNum=0, Ns_FrameType=CAN, Ns_FrameBufferSize=0, Ns_OverflowCntOutFlg=off, Ns_SampleTime=-1}
      | uint16(Ns_DeviceID),
      | uint16(Ns_ChannelNum),
      | uint16(Ns_FrameType),
      | uint16(Ns_FrameBufferSize),
      | uint8(Ns_OverflowCntOutFlg),
      | double(Ns_SampleTime)
      mask prompts: Ns_DeviceID "Device:"; Ns_ChannelNum "Channel number:"; Ns_FrameType "Frame type:"; Ns_FrameBufferSize "Frame buffer size:"; Ns_OverflowCntOutFlg "Overflow count output"; Ns_SampleTime "Sample time:"
      mask init:
      | NSTC297CANTransmit_callback('portlabels');
      mask TypeOptions Ns_DeviceID: General Control Unit Gen2 | ADAS Control Unit Gen2
      mask TypeOptions Ns_ChannelNum: 0 | 1 | 2 | 3 | 4 | 5
      mask TypeOptions Ns_FrameType: CAN | CANFD
      mask Display: color('blue');text(0.98,0.9,'NovSteeds TC297','horizontalAlignment','right');color('blue');text(0.5,0.65,'CAN Transmit','horizontalAlignment','center');color('black');text(0.5,0.35,'Type: CAN','horizontalAlignment','center');text(0.5,0.50,'Channel: 0','horizontalAlignment','center');port_label('input',1, 'Msg');
  S-Function3 : S-Function  FunctionName=NSTC297CANTransmitBlkLib  Parameters=|  SFunctionDeploymentMode=off  EnableBusSupport=off  mask(NSTC297 CAN Transmit){Ns_DeviceID=General Control Unit Gen2, Ns_ChannelNum=0, Ns_FrameType=CAN, Ns_FrameBufferSize=0, Ns_OverflowCntOutFlg=off, Ns_SampleTime=-1}
      | uint16(Ns_DeviceID),
      | uint16(Ns_ChannelNum),
      | uint16(Ns_FrameType),
      | uint16(Ns_FrameBufferSize),
      | uint8(Ns_OverflowCntOutFlg),
      | double(Ns_SampleTime)
      mask prompts: Ns_DeviceID "Device:"; Ns_ChannelNum "Channel number:"; Ns_FrameType "Frame type:"; Ns_FrameBufferSize "Frame buffer size:"; Ns_OverflowCntOutFlg "Overflow count output"; Ns_SampleTime "Sample time:"
      mask init:
      | NSTC297CANTransmit_callback('portlabels');
      mask TypeOptions Ns_DeviceID: General Control Unit Gen2 | ADAS Control Unit Gen2
      mask TypeOptions Ns_ChannelNum: 0 | 1 | 2 | 3 | 4 | 5
      mask TypeOptions Ns_FrameType: CAN | CANFD
      mask Display: color('blue');text(0.98,0.9,'NovSteeds TC297','horizontalAlignment','right');color('blue');text(0.5,0.65,'CAN Transmit','horizontalAlignment','center');color('black');text(0.5,0.35,'Type: CAN','horizontalAlignment','center');text(0.5,0.50,'Channel: 0','horizontalAlignment','center');port_label('input',1, 'Msg');
  S-Function4 : S-Function  FunctionName=NSTC297CANTransmitBlkLib  Parameters=|  SFunctionDeploymentMode=off  EnableBusSupport=off  mask(NSTC297 CAN Transmit){Ns_DeviceID=General Control Unit Gen2, Ns_ChannelNum=0, Ns_FrameType=CAN, Ns_FrameBufferSize=0, Ns_OverflowCntOutFlg=off, Ns_SampleTime=-1}
      | uint16(Ns_DeviceID),
      | uint16(Ns_ChannelNum),
      | uint16(Ns_FrameType),
      | uint16(Ns_FrameBufferSize),
      | uint8(Ns_OverflowCntOutFlg),
      | double(Ns_SampleTime)
      mask prompts: Ns_DeviceID "Device:"; Ns_ChannelNum "Channel number:"; Ns_FrameType "Frame type:"; Ns_FrameBufferSize "Frame buffer size:"; Ns_OverflowCntOutFlg "Overflow count output"; Ns_SampleTime "Sample time:"
      mask init:
      | NSTC297CANTransmit_callback('portlabels');
      mask TypeOptions Ns_DeviceID: General Control Unit Gen2 | ADAS Control Unit Gen2
      mask TypeOptions Ns_ChannelNum: 0 | 1 | 2 | 3 | 4 | 5
      mask TypeOptions Ns_FrameType: CAN | CANFD
      mask Display: color('blue');text(0.98,0.9,'NovSteeds TC297','horizontalAlignment','right');color('blue');text(0.5,0.65,'CAN Transmit','horizontalAlignment','center');color('black');text(0.5,0.35,'Type: CAN','horizontalAlignment','center');text(0.5,0.50,'Channel: 0','horizontalAlignment','center');port_label('input',1, 'Msg');
  S-Function5 : S-Function  FunctionName=NSTC297CANTransmitBlkLib  Parameters=|  SFunctionDeploymentMode=off  EnableBusSupport=off  mask(NSTC297 CAN Transmit){Ns_DeviceID=General Control Unit Gen2, Ns_ChannelNum=0, Ns_FrameType=CAN, Ns_FrameBufferSize=0, Ns_OverflowCntOutFlg=off, Ns_SampleTime=-1}
      | uint16(Ns_DeviceID),
      | uint16(Ns_ChannelNum),
      | uint16(Ns_FrameType),
      | uint16(Ns_FrameBufferSize),
      | uint8(Ns_OverflowCntOutFlg),
      | double(Ns_SampleTime)
      mask prompts: Ns_DeviceID "Device:"; Ns_ChannelNum "Channel number:"; Ns_FrameType "Frame type:"; Ns_FrameBufferSize "Frame buffer size:"; Ns_OverflowCntOutFlg "Overflow count output"; Ns_SampleTime "Sample time:"
      mask init:
      | NSTC297CANTransmit_callback('portlabels');
      mask TypeOptions Ns_DeviceID: General Control Unit Gen2 | ADAS Control Unit Gen2
      mask TypeOptions Ns_ChannelNum: 0 | 1 | 2 | 3 | 4 | 5
      mask TypeOptions Ns_FrameType: CAN | CANFD
      mask Display: color('blue');text(0.98,0.9,'NovSteeds TC297','horizontalAlignment','right');color('blue');text(0.5,0.65,'CAN Transmit','horizontalAlignment','center');color('black');text(0.5,0.35,'Type: CAN','horizontalAlignment','center');text(0.5,0.50,'Channel: 0','horizontalAlignment','center');port_label('input',1, 'Msg');
  S-Function8 : S-Function  FunctionName=NSTC297CANTransmitBlkLib  Parameters=|  SFunctionDeploymentMode=off  EnableBusSupport=off  mask(NSTC297 CAN Transmit){Ns_DeviceID=General Control Unit Gen2, Ns_ChannelNum=0, Ns_FrameType=CAN, Ns_FrameBufferSize=0, Ns_OverflowCntOutFlg=off, Ns_SampleTime=-1}
      | uint16(Ns_DeviceID),
      | uint16(Ns_ChannelNum),
      | uint16(Ns_FrameType),
      | uint16(Ns_FrameBufferSize),
      | uint8(Ns_OverflowCntOutFlg),
      | double(Ns_SampleTime)
      mask prompts: Ns_DeviceID "Device:"; Ns_ChannelNum "Channel number:"; Ns_FrameType "Frame type:"; Ns_FrameBufferSize "Frame buffer size:"; Ns_OverflowCntOutFlg "Overflow count output"; Ns_SampleTime "Sample time:"
      mask init:
      | NSTC297CANTransmit_callback('portlabels');
      mask TypeOptions Ns_DeviceID: General Control Unit Gen2 | ADAS Control Unit Gen2
      mask TypeOptions Ns_ChannelNum: 0 | 1 | 2 | 3 | 4 | 5
      mask TypeOptions Ns_FrameType: CAN | CANFD
      mask Display: color('blue');text(0.98,0.9,'NovSteeds TC297','horizontalAlignment','right');color('blue');text(0.5,0.65,'CAN Transmit','horizontalAlignment','center');color('black');text(0.5,0.35,'Type: CAN','horizontalAlignment','center');text(0.5,0.50,'Channel: 0','horizontalAlignment','center');port_label('input',1, 'Msg');
  S-Function9 : S-Function  FunctionName=NSTC297CANTransmitBlkLib  Parameters=|  SFunctionDeploymentMode=off  EnableBusSupport=off  mask(NSTC297 CAN Transmit){Ns_DeviceID=General Control Unit Gen2, Ns_ChannelNum=0, Ns_FrameType=CAN, Ns_FrameBufferSize=0, Ns_OverflowCntOutFlg=off, Ns_SampleTime=-1}
      | uint16(Ns_DeviceID),
      | uint16(Ns_ChannelNum),
      | uint16(Ns_FrameType),
      | uint16(Ns_FrameBufferSize),
      | uint8(Ns_OverflowCntOutFlg),
      | double(Ns_SampleTime)
      mask prompts: Ns_DeviceID "Device:"; Ns_ChannelNum "Channel number:"; Ns_FrameType "Frame type:"; Ns_FrameBufferSize "Frame buffer size:"; Ns_OverflowCntOutFlg "Overflow count output"; Ns_SampleTime "Sample time:"
      mask init:
      | NSTC297CANTransmit_callback('portlabels');
      mask TypeOptions Ns_DeviceID: General Control Unit Gen2 | ADAS Control Unit Gen2
      mask TypeOptions Ns_ChannelNum: 0 | 1 | 2 | 3 | 4 | 5
      mask TypeOptions Ns_FrameType: CAN | CANFD
      mask Display: color('blue');text(0.98,0.9,'NovSteeds TC297','horizontalAlignment','right');color('blue');text(0.5,0.65,'CAN Transmit','horizontalAlignment','center');color('black');text(0.5,0.35,'Type: CAN','horizontalAlignment','center');text(0.5,0.50,'Channel: 0','horizontalAlignment','center');port_label('input',1, 'Msg');
  wires:
  <FRRdr>/1 -> Bus Selector1/1
  Bus Selector1/3 -> Bus Selector2/1  "<M10ObjInfo>"
  Bus Selector1/4 -> Bus Selector5/1  "<M11ObjInfo>"
  Bus Selector1/2 -> Bus Selector4/1  "<M01ObjInfo>"
  Bus Selector1/1 -> Bus Selector3/1  "<M00ObjInfo>"
  CAN Pack2/1 -> S-Function1/1
  CAN Pack1/1 -> S-Function8/1
  Bus Selector3/1 -> CAN Pack1/1  "<Id_S0_001>"
  Bus Selector3/2 -> CAN Pack1/2  "<XPos_S0_001>"
  Bus Selector3/3 -> CAN Pack1/3  "<YPos_S0_001>"
  Bus Selector3/4 -> CAN Pack1/4  "<XVelocity_S0_001>"
  Bus Selector3/5 -> CAN Pack2/1  "<YVelocity_S0_001>"
  Bus Selector3/6 -> CAN Pack2/2  "<XAcc_S0_001>"
  Bus Selector3/7 -> CAN Pack2/3  "<YAcc_S0_001>"
  Bus Selector4/7 -> CAN Pack4/3  "<YAcc_S0_002>"
  Bus Selector4/6 -> CAN Pack4/2  "<XAcc_S0_002>"
  Bus Selector4/5 -> CAN Pack4/1  "<YVelocity_S0_002>"
  Bus Selector4/4 -> CAN Pack3/4  "<XVelocity_S0_002>"
  Bus Selector4/3 -> CAN Pack3/3  "<YPos_S0_002>"
  Bus Selector4/2 -> CAN Pack3/2  "<XPos_S0_002>"
  Bus Selector4/1 -> CAN Pack3/1  "<Id_S0_002>"
  CAN Pack3/1 -> S-Function3/1
  CAN Pack4/1 -> S-Function2/1
  CAN Pack6/1 -> S-Function4/1
  CAN Pack5/1 -> S-Function5/1
  Bus Selector2/1 -> CAN Pack5/1  "<Id_S0_003>"
  Bus Selector2/2 -> CAN Pack5/2  "<XPos_S0_003>"
  Bus Selector2/3 -> CAN Pack5/3  "<YPos_S0_003>"
  Bus Selector2/4 -> CAN Pack5/4  "<XVelocity_S0_003>"
  Bus Selector2/5 -> CAN Pack6/1  "<YVelocity_S0_003>"
  Bus Selector2/6 -> CAN Pack6/2  "<XAcc_S0_003>"
  Bus Selector2/7 -> CAN Pack6/3  "<YAcc_S0_003>"
  CAN Pack10/1 -> S-Function9/1
  CAN Pack9/1 -> S-Function10/1
  Bus Selector5/2 -> CAN Pack9/2  "<XPos_S0_004>"
  Bus Selector5/3 -> CAN Pack9/3  "<YPos_S0_004>"
  Bus Selector5/4 -> CAN Pack9/4  "<XVelocity_S0_004>"
  Bus Selector5/5 -> CAN Pack10/1  "<YVelocity_S0_004>"
  Bus Selector5/6 -> CAN Pack10/2  "<XAcc_S0_004>"
  Bus Selector5/7 -> CAN Pack10/3  "<YAcc_S0_004>"
  Bus Selector5/1 -> CAN Pack9/1  "<Id_S0_004>"
